simulink model "FMS22"  (R2018b)
settings: configuration reference "fms_config" (kept outside this file)
values from neighbouring files (symbols this model uses):
  FMS_EXPORT = Simulink.Parameter(FMS_EXPORT_VALUE)    [fms_model_init.m]
  FMS_PARAM = Simulink.Parameter(FMS_PARAM_VALUE)    [fms_model_init.m]
undefined symbols (not defined in the file or in its folder): actuator_cmd, ControlMode, ctrl_mode, DiscIntNeverNeededParam, mode, p_cmd, phi_cmd, psi_rate_cmd, q_cmd, r_cmd, reset, status, theta_cmd, throttle_cmd, u_cmd, v_cmd, VehicleMode, VehicleStatus, w_cmd
libraries: FMT_Model_Lib x18, simulink x16
(part 1 of 4)
settings Model: Creator=jiachi  LastModifiedBy=jiachi
settings ConfigSetRef: SourceLocation=Base Workspace

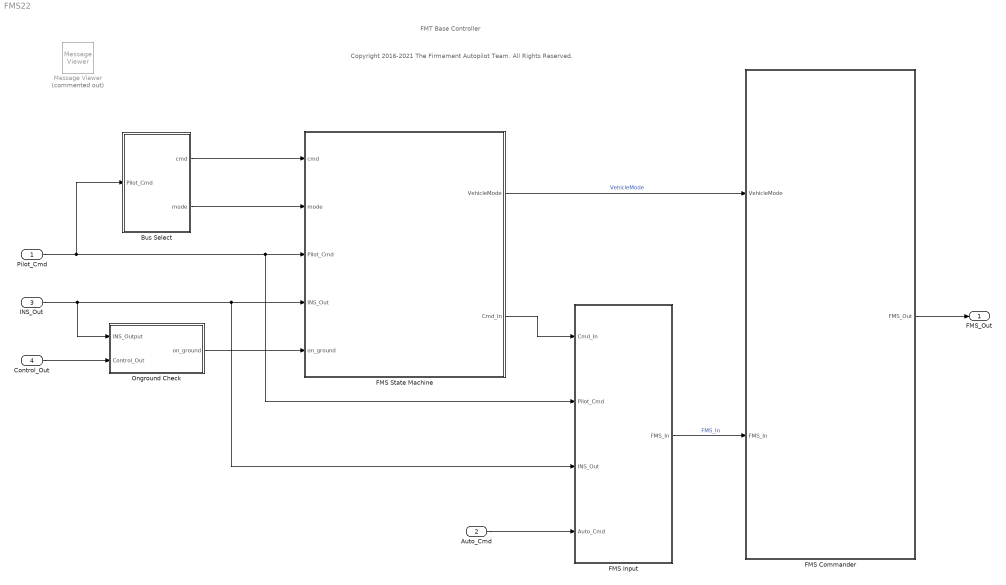
== system FMS22 ==
  note: FMT Base Controller
  note: Copyright 2016-2021 The Firmament Autopilot Team. All Rights Reserved.
  Pilot_Cmd : Inport  OutDataTypeStr=Bus: Pilot_Cmd_Bus
  Auto_Cmd : Inport  Port=2  OutDataTypeStr=Bus: Auto_Cmd_Bus
  INS_Out : Inport  Port=3  OutDataTypeStr=Bus: INS_Out_Bus
  Control_Out : Inport  Port=4  OutDataTypeStr=Bus: Control_Out_Bus
  Bus Select : Subsystem
  FMS Commander : Subsystem  TreatAsAtomicUnit=on
  FMS Input : Subsystem  TreatAsAtomicUnit=on
  FMS State Machine : Stateflow chart  TreatAsAtomicUnit=on
  Message Viewer : MessageViewer  Commented=on  SavedRootId=#
  Onground Check : Subsystem
  FMS_Out : Outport  OutDataTypeStr=Bus: FMS_Out_Bus
  wires:
  Pilot_Cmd/1 -> FMS State Machine/3(Pilot_Cmd), FMS Input/2(Pilot_Cmd), Bus Select/1(Pilot_Cmd)
  INS_Out/1 -> FMS Input/3(INS_Out), FMS State Machine/4(INS_Out), Onground Check/1(INS_Output)
  Control_Out/1 -> Onground Check/2(Control_Out)
  Onground Check/1(on_ground) -> FMS State Machine/5(on_ground)
  FMS State Machine/1(" VehicleMode") -> FMS Commander/1(VehicleMode)  "VehicleMode"
  FMS Input/1(FMS_In) -> FMS Commander/2(FMS_In)  "FMS_In"
  Auto_Cmd/1 -> FMS Input/4(Auto_Cmd)
  FMS Commander/1(FMS_Out) -> FMS_Out/1
  FMS State Machine/2(Cmd_In) -> FMS Input/1(Cmd_In)
  Bus Select/1(cmd) -> FMS State Machine/1(cmd)
  Bus Select/2(mode) -> FMS State Machine/2(mode)

== system FMS22/Bus Select ==
  Pilot_Cmd : Inport
  Bus Selector : BusSelector  OutputSignals=cmd_1,mode
  Data Type Conversion : DataTypeConversion  OutDataTypeStr=Enum: FMS_Cmd
  Data Type Conversion1 : DataTypeConversion  OutDataTypeStr=Enum: PilotMode
  cmd : Outport
  mode : Outport  Port=2
  wires:
  Data Type Conversion1/1 -> mode/1
  Pilot_Cmd/1 -> Bus Selector/1
  Bus Selector/1 -> Data Type Conversion/1  "<cmd_1>"
  Bus Selector/2 -> Data Type Conversion1/1  "<mode>"
  Data Type Conversion/1 -> cmd/1

== system FMS22/FMS Commander ==
  In Bus Element1 : Inport  PortName=VehicleMode
  In Bus Element2 : Inport  PortName=VehicleMode
  In Bus Element : Inport  Port=2  PortName=FMS_In
  Arm : Subsystem  TreatAsAtomicUnit=on
  Bus Assignment : BusAssignment  AssignedSignals=timestamp
  Disarm : Subsystem  TreatAsAtomicUnit=on
  Merge : Merge  Inputs=3
  Standby : Subsystem  TreatAsAtomicUnit=on
  Switch Case : SwitchCase  CaseConditions={[VehicleMode.Disarm,VehicleMode.None], VehicleMode.Standby}
  timestamp : Subsystem  mask{sample_time=FMS_EXPORT.period}
      mask prompts: sample_time "sample time (ms)"
  FMS_Out : Outport
  wires:
  Switch Case/1 -> Disarm/Action
  Merge/1 -> Bus Assignment/1
  Switch Case/2 -> Standby/Action
  Switch Case/3 -> Arm/Action
  Disarm/1(FMS_Out) -> Merge/1
  Standby/1(FMS_Out) -> Merge/2
  Arm/1(FMS_Out) -> Merge/3
  In Bus Element/1 -> Arm/2(FMS_In)
  In Bus Element1/1 -> Switch Case/1
  In Bus Element2/1 -> Arm/1(VehicleMode)
  timestamp/1(timestamp_ms) -> Bus Assignment/2
  Bus Assignment/1 -> FMS_Out/1

== system FMS22/FMS Input ==
  Cmd_In : Inport
  Pilot_Cmd : Inport  Port=2
  INS_Out : Inport  Port=3
  Auto_Cmd : Inport  Port=4
  Bus Creator : BusCreator  Inputs=4
  Signal Copy{,1..3} (4 alike) : SignalConversion  OverrideOpt=off
  FMS_In : Outport
  wires:
  Bus Creator/1 -> FMS_In/1
  Pilot_Cmd/1 -> Signal Copy2/1
  Auto_Cmd/1 -> Signal Copy/1
  INS_Out/1 -> Signal Copy1/1
  Signal Copy2/1 -> Bus Creator/1  "Pilot_Cmd"
  Signal Copy/1 -> Bus Creator/2  "Auto_Cmd"
  Signal Copy1/1 -> Bus Creator/3  "INS_Out"
  Cmd_In/1 -> Signal Copy3/1
  Signal Copy3/1 -> Bus Creator/4  "Cmd_In"

== system FMS22/Onground Check ==
  INS_Output : Inport
  Control_Out : Inport  Port=2
  Bus Selector1 : BusSelector  OutputSignals=actuator_cmd
  Bus Selector3 : BusSelector  OutputSignals=ax,ay,az
  Compare To Constant : simulink/Logic and Bit Operations/Compare To Constant  relop=<  const=1200  OutDataTypeStr=boolean
  Constant : Constant  Value=4  OutDataTypeStr=uint16
  Divide : Product  Inputs=*/
  First Order LPF : FMT_Model_Lib/Filter/First Order LPF  fc=1/(2*pi*0.5)
      settings: SourceProductName=FMT Toolbox
  First Order LPF2 : FMT_Model_Lib/Filter/First Order LPF  fc=1/(2*pi*0.1)
      settings: SourceProductName=FMT Toolbox
  Interval Test : simulink/Logic and Bit Operations/Interval Test  IntervalClosedRight=on  uplimit=[0.5, 0.5, -9.806+0.5]  IntervalClosedLeft=on  lowlimit=[-0.5, -0.5, -9.806-0.5]  OutDataTypeStr=boolean
  Logical Operator : Logic  Inputs=1  AllPortsSameDT=off  OutDataTypeStr=boolean
  Logical Operator1 : Logic  AllPortsSameDT=off  OutDataTypeStr=boolean
  Matrix Concatenate3 : Concatenate  NumInputs=3  ConcatenateDimension=2
  Selector : Selector  InputPortWidth=16  IndexOptions=Index vector (dialog)  Indices=[1:4]  OutputSizes=1
  Sum of Elements : Sum  Inputs=+
  on_ground : Outport
  wires:
  Bus Selector3/2 -> Matrix Concatenate3/2  "<ay>"
  Compare To Constant/1 -> Logical Operator1/2
  Bus Selector3/3 -> Matrix Concatenate3/3  "<az>"
  Bus Selector1/1 -> Selector/1  "<actuator_cmd>"
  Bus Selector3/1 -> Matrix Concatenate3/1  "<ax>"
  Selector/1 -> Sum of Elements/1
  INS_Output/1 -> Bus Selector3/1
  Control_Out/1 -> Bus Selector1/1
  Matrix Concatenate3/1 -> First Order LPF/1
  Interval Test/1 -> Logical Operator/1
  Sum of Elements/1 -> Divide/1
  Constant/1 -> Divide/2
  First Order LPF/1 -> Interval Test/1
  Divide/1 -> First Order LPF2/1
  First Order LPF2/1 -> Compare To Constant/1
  Logical Operator/1 -> Logical Operator1/1
  Logical Operator1/1 -> on_ground/1

== system FMS22/FMS Commander/Arm ==
  In Bus Element{2..5} (4 alike) : Inport  PortName=VehicleMode
  In Bus Element{,1,6..7} (4 alike) : Inport  Port=2  PortName=FMS_In
  Action Port : ActionPort  InitializeStates=reset  ActionType=default
  Assist : Subsystem  TreatAsAtomicUnit=on
  Auto : Subsystem  TreatAsAtomicUnit=on
  Manual : Subsystem  TreatAsAtomicUnit=on
  Merge : Merge  Inputs=4
  SubMode : Subsystem  TreatAsAtomicUnit=on
  Switch Case : SwitchCase  CaseConditions={[VehicleMode.Land,VehicleMode.Return,VehicleMode.Takeoff,VehicleMode.Hold], [VehicleMode.Offboard,VehicleMode.Mission],[VehicleMode.Acro,VehicleMode.Stabilize,VehicleMode.Altitude,VehicleMode.Position],VehicleMode.Manual}  ShowDefaultCase=off
  FMS_Out : Outport
  wires:
  Merge/1 -> FMS_Out/1
  Switch Case/1 -> SubMode/Action
  Switch Case/2 -> Auto/Action
  Switch Case/3 -> Assist/Action
  Switch Case/4 -> Manual/Action
  SubMode/1(FMS_Out) -> Merge/1
  Auto/1(FMS_Out) -> Merge/2
  Assist/1(FMS_Out) -> Merge/3
  Manual/1(FMS_Out) -> Merge/4
  In Bus Element/1 -> SubMode/2(FMS_In)
  In Bus Element1/1 -> Assist/2(FMS_In)
  In Bus Element2/1 -> Switch Case/1
  In Bus Element3/1 -> SubMode/1(VehicleMode)
  In Bus Element4/1 -> Assist/1(VehicleMode)
  In Bus Element5/1 -> Auto/1(VehicleMode)
  In Bus Element6/1 -> Auto/2(FMS_In)
  In Bus Element7/1 -> Manual/1(FMS_In)

== system FMS22/FMS Commander/Disarm ==
  Action Port : ActionPort  InitializeStates=reset  ActionType=case
  Bus Assignment : BusAssignment  AssignedSignals=reset,status,mode,actuator_cmd
  Constant : Constant  Value=0  OutDataTypeStr=Bus: FMS_Out_Bus
  Constant1 : Constant  Value=VehicleStatus.Disarm
  Constant2 : Constant  OutDataTypeStr=Inherit: Inherit via back propagation
  Constant3 : Constant  Value=[1000;1000;1000;1000]  VectorParams1D=off  OutDataTypeStr=Inherit: Inherit via back propagation
  Constant4 : Constant  Value=zeros(12,1)  OutDataTypeStr=Inherit: Inherit via back propagation
  Constant5 : Constant  Value=VehicleMode.Disarm
  Data Type Conversion : DataTypeConversion
  Data Type Conversion1 : DataTypeConversion
  Mux : Mux  Inputs=2
  FMS_Out : Outport
  wires:
  Mux/1 -> Bus Assignment/5
  Constant4/1 -> Mux/2
  Constant3/1 -> Mux/1
  Constant1/1 -> Data Type Conversion/1
  Constant2/1 -> Bus Assignment/2
  Bus Assignment/1 -> FMS_Out/1
  Constant/1 -> Bus Assignment/1
  Constant5/1 -> Data Type Conversion1/1
  Data Type Conversion/1 -> Bus Assignment/3
  Data Type Conversion1/1 -> Bus Assignment/4

== system FMS22/FMS Commander/Standby ==
  Action Port : ActionPort  InitializeStates=reset  ActionType=case
  Bus Assignment : BusAssignment  AssignedSignals=reset,status,mode,actuator_cmd
  Constant : Constant  Value=0  OutDataTypeStr=Bus: FMS_Out_Bus
  Constant1 : Constant  Value=VehicleStatus.Standby
  Constant2 : Constant  OutDataTypeStr=Inherit: Inherit via back propagation
  Constant3 : Constant  Value=[1150;1150;1150;1150]  VectorParams1D=off  OutDataTypeStr=Inherit: Inherit via back propagation
  Constant4 : Constant  Value=zeros(12,1)  OutDataTypeStr=Inherit: Inherit via back propagation
  Constant5 : Constant  Value=VehicleMode.Standby
  Data Type Conversion1 : DataTypeConversion
  Data Type Conversion2 : DataTypeConversion
  Mux : Mux  Inputs=2
  FMS_Out : Outport
  wires:
  Constant/1 -> Bus Assignment/1
  Bus Assignment/1 -> FMS_Out/1
  Constant2/1 -> Bus Assignment/2
  Constant1/1 -> Data Type Conversion2/1
  Constant3/1 -> Mux/1
  Constant4/1 -> Mux/2
  Constant5/1 -> Data Type Conversion1/1
  Data Type Conversion2/1 -> Bus Assignment/3
  Mux/1 -> Bus Assignment/5
  Data Type Conversion1/1 -> Bus Assignment/4

== system FMS22/FMS Commander/timestamp ==
  Constant : Constant  Value=sample_time
  Data Type Conversion : DataTypeConversion  OutDataTypeStr=uint32
  Discrete-Time Integrator : DiscreteIntegrator  IntegratorMethod=Accumulation: Forward Euler  SampleTime=-1  ICPrevOutput=DiscIntNeverNeededParam  ICPrevScaledInput=DiscIntNeverNeededParam
  timestamp_ms : Outport
  wires:
  Discrete-Time Integrator/1 -> Data Type Conversion/1
  Constant/1 -> Discrete-Time Integrator/1
  Data Type Conversion/1 -> timestamp_ms/1

== system FMS22/FMS Commander/Arm/Assist ==
  VehicleMode : Inport
  In Bus Element{1..4} (4 alike) : Inport  Port=2  PortName=FMS_In
  Action Port : ActionPort  InitializeStates=reset  ActionType=case
  Acro : Subsystem
      settings: UndoDeleteFcn=Stateflow.SLINSF.SimulinkMan.restorePreDeleteFcn  PreDeleteFcn=Stateflow.SLINSF.SimulinkMan.removePreDeleteFcn
  Altitude : Subsystem
      settings: UndoDeleteFcn=Stateflow.SLINSF.SimulinkMan.restorePreDeleteFcn  PreDeleteFcn=Stateflow.SLINSF.SimulinkMan.removePreDeleteFcn
  Merge : Merge  Inputs=4
  Position : Subsystem
      settings: UndoDeleteFcn=Stateflow.SLINSF.SimulinkMan.restorePreDeleteFcn  PreDeleteFcn=Stateflow.SLINSF.SimulinkMan.removePreDeleteFcn
  Stabilize : Subsystem
      settings: UndoDeleteFcn=Stateflow.SLINSF.SimulinkMan.restorePreDeleteFcn  PreDeleteFcn=Stateflow.SLINSF.SimulinkMan.removePreDeleteFcn
  Switch Case : SwitchCase  CaseConditions={VehicleMode.Acro,VehicleMode.Stabilize,VehicleMode.Altitude,VehicleMode.Position}  ShowDefaultCase=off
  FMS_Out : Outport
  wires:
  VehicleMode/1 -> Switch Case/1
  In Bus Element1/1 -> Position/1(FMS_In)
  Switch Case/4 -> Position/Action
  Switch Case/3 -> Altitude/Action
  In Bus Element2/1 -> Altitude/1(FMS_In)
  Switch Case/2 -> Stabilize/Action
  In Bus Element3/1 -> Stabilize/1(FMS_In)
  In Bus Element4/1 -> Acro/1(FMS_In)
  Switch Case/1 -> Acro/Action
  Acro/1(FMS_Out) -> Merge/1
  Stabilize/1(FMS_Out) -> Merge/2
  Altitude/1(FMS_Out) -> Merge/3
  Position/1(FMS_Out) -> Merge/4
  Merge/1 -> FMS_Out/1

== system FMS22/FMS Commander/Arm/Auto ==
  In Bus Element5 : Inport  PortName=VehicleMode
  In Bus Element6 : Inport  Port=2  PortName=FMS_In
  In Bus Element1 : Inport  Port=2  PortName=FMS_In
  Action Port : ActionPort  InitializeStates=reset  ActionType=case
  Merge : Merge
  Mission : Subsystem
      settings: UndoDeleteFcn=Stateflow.SLINSF.SimulinkMan.restorePreDeleteFcn  PreDeleteFcn=Stateflow.SLINSF.SimulinkMan.removePreDeleteFcn
  Offboard : Subsystem
      settings: UndoDeleteFcn=Stateflow.SLINSF.SimulinkMan.restorePreDeleteFcn  PreDeleteFcn=Stateflow.SLINSF.SimulinkMan.removePreDeleteFcn
  Switch Case : SwitchCase  CaseConditions={VehicleMode.Offboard,VehicleMode.Mission}  ShowDefaultCase=off
  FMS_Out : Outport
  wires:
  Merge/1 -> FMS_Out/1
  In Bus Element5/1 -> Switch Case/1
  In Bus Element6/1 -> Offboard/1(FMS_In)
  Switch Case/1 -> Offboard/Action
  In Bus Element1/1 -> Mission/1(FMS_In)
  Switch Case/2 -> Mission/Action
  Offboard/1(FMS_Out) -> Merge/1
  Mission/1(FMS_Out) -> Merge/2

== system FMS22/FMS Commander/Arm/Manual ==
  In Bus Element7 : Inport  PortName=FMS_In
  Action Port : ActionPort  InitializeStates=reset  ActionType=case
  Bus Assignment : BusAssignment  AssignedSignals=reset,status,mode
  Constant : Constant  Value=0  OutDataTypeStr=Bus: FMS_Out_Bus
  Constant1 : Constant  Value=VehicleStatus.Disarm
  Constant2 : Constant  OutDataTypeStr=Inherit: Inherit via back propagation
  Constant5 : Constant  Value=VehicleMode.Manual
  Data Type Conversion : DataTypeConversion
  Data Type Conversion1 : DataTypeConversion
  Terminator : Terminator
  FMS_Out : Outport
  wires:
  Data Type Conversion1/1 -> Bus Assignment/4
  Data Type Conversion/1 -> Bus Assignment/3
  Constant5/1 -> Data Type Conversion1/1
  Constant/1 -> Bus Assignment/1
  Bus Assignment/1 -> FMS_Out/1
  Constant2/1 -> Bus Assignment/2
  Constant1/1 -> Data Type Conversion/1
  In Bus Element7/1 -> Terminator/1

== system FMS22/FMS Commander/Arm/SubMode ==
  In Bus Element : Inport  PortName=VehicleMode
  In Bus Element{1..4} (4 alike) : Inport  Port=2  PortName=FMS_In
  Action Port : ActionPort  InitializeStates=reset  ActionType=case
  Hold : Subsystem
      settings: UndoDeleteFcn=Stateflow.SLINSF.SimulinkMan.restorePreDeleteFcn  PreDeleteFcn=Stateflow.SLINSF.SimulinkMan.removePreDeleteFcn
  Land : Subsystem
      settings: UndoDeleteFcn=Stateflow.SLINSF.SimulinkMan.restorePreDeleteFcn  PreDeleteFcn=Stateflow.SLINSF.SimulinkMan.removePreDeleteFcn
  Merge : Merge  Inputs=4
  Return : Subsystem
      settings: UndoDeleteFcn=Stateflow.SLINSF.SimulinkMan.restorePreDeleteFcn  PreDeleteFcn=Stateflow.SLINSF.SimulinkMan.removePreDeleteFcn
  Switch Case : SwitchCase  CaseConditions={VehicleMode.Takeoff, VehicleMode.Land, VehicleMode.Return,VehicleMode.Hold}  ShowDefaultCase=off
  Takeoff : Subsystem
      settings: UndoDeleteFcn=Stateflow.SLINSF.SimulinkMan.restorePreDeleteFcn  PreDeleteFcn=Stateflow.SLINSF.SimulinkMan.removePreDeleteFcn
  FMS_Out : Outport
  wires:
  Merge/1 -> FMS_Out/1
  In Bus Element/1 -> Switch Case/1
  In Bus Element1/1 -> Land/1(FMS_In)
  Land/1(FMS_Out) -> Merge/2
  Switch Case/2 -> Land/Action
  Switch Case/1 -> Takeoff/Action
  In Bus Element2/1 -> Takeoff/1(FMS_In)
  Takeoff/1(FMS_Out) -> Merge/1
  Switch Case/3 -> Return/Action
  In Bus Element3/1 -> Return/1(FMS_In)
  Return/1(FMS_Out) -> Merge/3
  Hold/1(FMS_Out) -> Merge/4
  In Bus Element4/1 -> Hold/1(FMS_In)
  Switch Case/4 -> Hold/Action

== system FMS22/FMS Commander/Arm/Assist/Acro ==
  FMS_In : Inport
  Action Port : ActionPort  InitializeStates=reset  ActionType=case
      settings: CopyFcn=Stateflow.SLINSF.SimulinkMan.removeBlockPreDeleteFcn
  Angular Rate Command : Subsystem
  Bus Assignment : BusAssignment  AssignedSignals=status,mode,ctrl_mode,p_cmd,q_cmd,r_cmd,throttle_cmd
  Constant : Constant  Value=0  OutDataTypeStr=Bus: FMS_Out_Bus
  Constant1 : Constant  Value=VehicleMode.Acro
  Constant2 : Constant  Value=ControlMode.Acro
  Constant5 : Constant  Value=VehicleStatus.Arm
  Data Type Conversion : DataTypeConversion
  Data Type Conversion1 : DataTypeConversion
  Data Type Conversion2 : DataTypeConversion
  Throttle Command : Subsystem
  FMS_Out : Outport
  wires:
  Data Type Conversion2/1 -> Bus Assignment/4
  Constant2/1 -> Data Type Conversion2/1
  Data Type Conversion1/1 -> Bus Assignment/3
  Constant1/1 -> Data Type Conversion1/1
  Data Type Conversion/1 -> Bus Assignment/2
  Bus Assignment/1 -> FMS_Out/1
  Throttle Command/1(throttle_cmd) -> Bus Assignment/8
  Constant/1 -> Bus Assignment/1
  Constant5/1 -> Data Type Conversion/1
  Angular Rate Command/1(p_cmd_radPs) -> Bus Assignment/5
  Angular Rate Command/2(q_cmd_radPs) -> Bus Assignment/6
  Angular Rate Command/3(r_cmd_radPs) -> Bus Assignment/7
  FMS_In/1 -> Throttle Command/1(FMS_In), Angular Rate Command/1(FMS_In)

== system FMS22/FMS Commander/Arm/Assist/Altitude ==
  In Bus Element1 : Inport  PortName=FMS_In
  Action Port : ActionPort  InitializeStates=reset  ActionType=case
      settings: CopyFcn=Stateflow.SLINSF.SimulinkMan.removeBlockPreDeleteFcn
  Altitude Command : Subsystem
  Attitude Command : Subsystem
  Bus Assignment : BusAssignment  AssignedSignals=status,mode,ctrl_mode,phi_cmd,theta_cmd,psi_rate_cmd,w_cmd
  Constant : Constant  Value=0  OutDataTypeStr=Bus: FMS_Out_Bus
  Constant1 : Constant  Value=VehicleMode.Altitude
  Constant2 : Constant  Value=ControlMode.ALTCTL
  Constant5 : Constant  Value=VehicleStatus.Arm
  Data Type Conversion1 : DataTypeConversion
  Data Type Conversion2 : DataTypeConversion
  Data Type Conversion3 : DataTypeConversion
  Heading Command : Subsystem
  FMS_Out : Outport
  wires:
  Constant5/1 -> Data Type Conversion1/1
  Constant/1 -> Bus Assignment/1
  Heading Command/1(psi_rate_cmd_radPs) -> Bus Assignment/7
  Altitude Command/1(w_cmd_mPs) -> Bus Assignment/8
  Attitude Command/1(phi_cmd_radPs) -> Bus Assignment/5
  Attitude Command/2(theta_cmd_radPs) -> Bus Assignment/6
  Bus Assignment/1 -> FMS_Out/1
  Data Type Conversion1/1 -> Bus Assignment/2
  Constant1/1 -> Data Type Conversion2/1
  Data Type Conversion2/1 -> Bus Assignment/3
  Data Type Conversion3/1 -> Bus Assignment/4
  Constant2/1 -> Data Type Conversion3/1
  In Bus Element1/1 -> Heading Command/1(FMS_In), Altitude Command/1(FMS_In), Attitude Command/1(FMS_In)

== system FMS22/FMS Commander/Arm/Assist/Position ==
  FMS_In : Inport
  Action Port : ActionPort  InitializeStates=reset  ActionType=case
      settings: CopyFcn=Stateflow.SLINSF.SimulinkMan.removeBlockPreDeleteFcn
  Altitude Command : Subsystem
  Bus Assignment : BusAssignment  AssignedSignals=status,mode,ctrl_mode,psi_rate_cmd,u_cmd,v_cmd,w_cmd
  Constant : Constant  Value=0  OutDataTypeStr=Bus: FMS_Out_Bus
  Constant1 : Constant  Value=VehicleMode.Position
  Constant2 : Constant  Value=ControlMode.POSCTL
  Constant5 : Constant  Value=VehicleStatus.Arm
  Data Type Conversion : DataTypeConversion
  Data Type Conversion1 : DataTypeConversion
  Data Type Conversion2 : DataTypeConversion
  Heading Command : Subsystem
  Position Command : Subsystem
  FMS_Out : Outport
  wires:
  Bus Assignment/1 -> FMS_Out/1
  Altitude Command/1(w_cmd_mPs) -> Bus Assignment/8
  Constant/1 -> Bus Assignment/1
  Position Command/1(u_cmd_mPs) -> Bus Assignment/6
  Constant5/1 -> Data Type Conversion/1
  Position Command/2(v_cmd_mPs) -> Bus Assignment/7
  Heading Command/1(psi_rate_cmd_radPs) -> Bus Assignment/5
  Data Type Conversion/1 -> Bus Assignment/2
  Constant1/1 -> Data Type Conversion1/1
  Data Type Conversion1/1 -> Bus Assignment/3
  Constant2/1 -> Data Type Conversion2/1
  Data Type Conversion2/1 -> Bus Assignment/4
  FMS_In/1 -> Heading Command/1(FMS_In), Altitude Command/1(FMS_In), Position Command/1(FMS_In)

== system FMS22/FMS Commander/Arm/Assist/Stabilize ==
  FMS_In : Inport
  Action Port : ActionPort  InitializeStates=reset  ActionType=case
      settings: CopyFcn=Stateflow.SLINSF.SimulinkMan.removeBlockPreDeleteFcn
  Attitude Command : Subsystem
  Bus Assignment : BusAssignment  AssignedSignals=status,mode,ctrl_mode,phi_cmd,theta_cmd,psi_rate_cmd,throttle_cmd
  Constant : Constant  Value=0  OutDataTypeStr=Bus: FMS_Out_Bus
  Constant1 : Constant  Value=VehicleMode.Stabilize
  Constant2 : Constant  Value=ControlMode.Stabilize
  Constant5 : Constant  Value=VehicleStatus.Arm
  Data Type Conversion : DataTypeConversion
  Data Type Conversion1 : DataTypeConversion
  Data Type Conversion2 : DataTypeConversion
  Heading Command : Subsystem
  Throttle Command : Subsystem
  FMS_Out : Outport
  wires:
  Constant5/1 -> Data Type Conversion/1
  Heading Command/1(psi_rate_cmd_radPs) -> Bus Assignment/7
  Constant/1 -> Bus Assignment/1
  Attitude Command/1(phi_cmd_radPs) -> Bus Assignment/5
  Throttle Command/1(throttle_cmd) -> Bus Assignment/8
  Attitude Command/2(theta_cmd_radPs) -> Bus Assignment/6
  FMS_In/1 -> Throttle Command/1(FMS_In), Heading Command/1(FMS_In), Attitude Command/1(FMS_In)
  Bus Assignment/1 -> FMS_Out/1
  Data Type Conversion/1 -> Bus Assignment/2
  Constant1/1 -> Data Type Conversion1/1
  Data Type Conversion1/1 -> Bus Assignment/3
  Constant2/1 -> Data Type Conversion2/1
  Data Type Conversion2/1 -> Bus Assignment/4

== system FMS22/FMS Commander/Arm/Auto/Mission ==
  FMS_In : Inport
  Action Port : ActionPort  InitializeStates=reset  ActionType=case
      settings: CopyFcn=Stateflow.SLINSF.SimulinkMan.removeBlockPreDeleteFcn
  Bus Assignment : BusAssignment  AssignedSignals=status,mode
  Constant : Constant  Value=0  OutDataTypeStr=Bus: FMS_Out_Bus
  Constant1 : Constant  Value=VehicleStatus.Disarm
  Constant2 : Constant  Value=VehicleMode.Mission
  Data Type Conversion : DataTypeConversion
  Data Type Conversion1 : DataTypeConversion
  Terminator : Terminator
  FMS_Out : Outport
  wires:
  Bus Assignment/1 -> FMS_Out/1
  Constant/1 -> Bus Assignment/1
  FMS_In/1 -> Terminator/1
  Constant1/1 -> Data Type Conversion/1
  Data Type Conversion/1 -> Bus Assignment/2
  Constant2/1 -> Data Type Conversion1/1
  Data Type Conversion1/1 -> Bus Assignment/3

== system FMS22/FMS Commander/Arm/Auto/Offboard ==
  FMS_In : Inport
  Action Port : ActionPort  InitializeStates=reset  ActionType=case
      settings: CopyFcn=Stateflow.SLINSF.SimulinkMan.removeBlockPreDeleteFcn
  Bus Assignment : BusAssignment  AssignedSignals=status,mode
  Constant : Constant  Value=0  OutDataTypeStr=Bus: FMS_Out_Bus
  Constant1 : Constant  Value=VehicleStatus.Disarm
  Constant2 : Constant  Value=VehicleMode.Offboard
  Data Type Conversion : DataTypeConversion
  Data Type Conversion1 : DataTypeConversion
  Terminator : Terminator
  FMS_Out : Outport
  wires:
  Bus Assignment/1 -> FMS_Out/1
  Constant/1 -> Bus Assignment/1
  FMS_In/1 -> Terminator/1
  Constant1/1 -> Data Type Conversion/1
  Data Type Conversion/1 -> Bus Assignment/2
  Constant2/1 -> Data Type Conversion1/1
  Data Type Conversion1/1 -> Bus Assignment/3

== system FMS22/FMS Commander/Arm/SubMode/Hold ==
  FMS_In : Inport
  Action Port : ActionPort  InitializeStates=reset  ActionType=case
      settings: CopyFcn=Stateflow.SLINSF.SimulinkMan.removeBlockPreDeleteFcn
  Altitude Command : Subsystem
  Bus Assignment : BusAssignment  AssignedSignals=status,mode,ctrl_mode,psi_rate_cmd,u_cmd,v_cmd,w_cmd
  Constant : Constant  Value=0  OutDataTypeStr=Bus: FMS_Out_Bus
  Constant1 : Constant  Value=VehicleMode.Hold
  Constant2 : Constant  Value=ControlMode.POSCTL
  Constant5 : Constant  Value=VehicleStatus.Arm
  Data Type Conversion : DataTypeConversion
  Data Type Conversion1 : DataTypeConversion
  Data Type Conversion2 : DataTypeConversion
  Heading Command : Subsystem
  Position Command : Subsystem
  FMS_Out : Outport
  wires:
  Bus Assignment/1 -> FMS_Out/1
  Altitude Command/1(w_cmd_mPs) -> Bus Assignment/8
  Constant/1 -> Bus Assignment/1
  Position Command/1(u_cmd_mPs) -> Bus Assignment/6
  Constant5/1 -> Data Type Conversion/1
  Position Command/2(v_cmd_mPs) -> Bus Assignment/7
  Heading Command/1(psi_rate_cmd_radPs) -> Bus Assignment/5
  Data Type Conversion/1 -> Bus Assignment/2
  Constant1/1 -> Data Type Conversion1/1
  Data Type Conversion1/1 -> Bus Assignment/3
  Constant2/1 -> Data Type Conversion2/1
  Data Type Conversion2/1 -> Bus Assignment/4
  FMS_In/1 -> Heading Command/1(FMS_In), Altitude Command/1(FMS_In), Position Command/1(FMS_In)

== system FMS22/FMS Commander/Arm/SubMode/Land ==
  FMS_In : Inport
  Action Port : ActionPort  InitializeStates=reset  ActionType=case
      settings: CopyFcn=Stateflow.SLINSF.SimulinkMan.removeBlockPreDeleteFcn
  Bus Assignment1 : BusAssignment  AssignedSignals=status,mode,ctrl_mode,psi_rate_cmd,u_cmd,v_cmd,w_cmd
  Bus Selector : BusSelector  OutputSignals=Cmd_In.p_land
  Constant : Constant  Value=0  OutDataTypeStr=Inherit: Inherit via back propagation
  Constant1 : Constant  Value=0  OutDataTypeStr=Bus: FMS_Out_Bus
  Constant2 : Constant  Value=ControlMode.POSCTL
  Constant3 : Constant  Value=VehicleMode.Land
  Constant4 : Constant  Value=0.5  OutDataTypeStr=Inherit: Inherit via back propagation
  Constant6 : Constant  Value=VehicleStatus.Arm
  Data Type Conversion : DataTypeConversion
  Data Type Conversion1 : DataTypeConversion
  Data Type Conversion2 : DataTypeConversion
  Position Command : Subsystem
  Reshape : Reshape  OutputDimensionality=Customize  OutputDimensions=[2,1]
  FMS_Out : Outport
  wires:
  Reshape/1 -> Position Command/2(land_xy_R)
  Bus Assignment1/1 -> FMS_Out/1
  Constant1/1 -> Bus Assignment1/1
  FMS_In/1 -> Position Command/1(FMS_In), Bus Selector/1
  Constant4/1 -> Bus Assignment1/8
  Position Command/1(u_cmd_mPs) -> Bus Assignment1/6
  Position Command/2(v_cmd_mPs) -> Bus Assignment1/7
  Constant/1 -> Bus Assignment1/5
  Constant2/1 -> Data Type Conversion2/1
  Constant6/1 -> Data Type Conversion/1
  Data Type Conversion/1 -> Bus Assignment1/2
  Constant3/1 -> Data Type Conversion1/1
  Data Type Conversion1/1 -> Bus Assignment1/3
  Data Type Conversion2/1 -> Bus Assignment1/4
  Bus Selector/1 -> Reshape/1  "<p_land>"

== system FMS22/FMS Commander/Arm/SubMode/Return ==
  FMS_In : Inport
  Action Port : ActionPort  InitializeStates=reset  ActionType=case
      settings: CopyFcn=Stateflow.SLINSF.SimulinkMan.removeBlockPreDeleteFcn
  Bus Assignment1 : BusAssignment  AssignedSignals=status,mode,ctrl_mode,u_cmd,v_cmd,w_cmd,psi_rate_cmd
  Bus Selector : BusSelector  OutputSignals=INS_Out
  Constant1 : Constant  Value=VehicleMode.Return
  Constant2 : Constant  Value=0  OutDataTypeStr=Bus: FMS_Out_Bus
  Constant3 : Constant  Value=ControlMode.POSCTL
  Constant6 : Constant  Value=VehicleStatus.Arm
  Coordinate Points : Subsystem
  Data Type Conversion : DataTypeConversion
  Data Type Conversion1 : DataTypeConversion
  Data Type Conversion2 : DataTypeConversion
  Heading Commander : Subsystem
  L1 : Constant  Value=10  OutDataTypeStr=single
  Sum : Sum  Inputs=+-|
  Velocity Commander : Subsystem
  FMS_Out : Outport
  wires:
  Sum/1 -> Heading Commander/2(p1p2)
  Velocity Commander/1(u_cmd) -> Bus Assignment1/5
  Coordinate Points/2(p2) -> Sum/1, Velocity Commander/2(p2)
  Coordinate Points/3(p3) -> Velocity Commander/3(p3)
  Velocity Commander/3(w_cmd) -> Bus Assignment1/7
  L1/1 -> Velocity Commander/4(L1)
  Velocity Commander/2(v_cmd) -> Bus Assignment1/6
  Constant3/1 -> Data Type Conversion2/1
  Coordinate Points/1(p1) -> Velocity Commander/1(p1), Sum/2
  Constant2/1 -> Bus Assignment1/1
  Heading Commander/1(psi_rad_cmd) -> Bus Assignment1/8
  Bus Assignment1/1 -> FMS_Out/1
  FMS_In/1 -> Bus Selector/1, Heading Commander/1(FMS_In), Coordinate Points/1(FMS_In)
  Data Type Conversion/1 -> Bus Assignment1/2
  Constant6/1 -> Data Type Conversion/1
  Data Type Conversion1/1 -> Bus Assignment1/3
  Data Type Conversion2/1 -> Bus Assignment1/4
  Constant1/1 -> Data Type Conversion1/1
  Bus Selector/1 -> Velocity Commander/5(INS_Out)  "<INS_Out>"

== system FMS22/FMS Commander/Arm/SubMode/Takeoff ==
  FMS_In : Inport
  Action Port : ActionPort  InitializeStates=reset  ActionType=case
      settings: CopyFcn=Stateflow.SLINSF.SimulinkMan.removeBlockPreDeleteFcn
  Bus Assignment1 : BusAssignment  AssignedSignals=status,mode,ctrl_mode,psi_rate_cmd,u_cmd,v_cmd,w_cmd
  Constant : Constant  Value=0  OutDataTypeStr=Inherit: Inherit via back propagation
  Constant1 : Constant  Value=0  OutDataTypeStr=Bus: FMS_Out_Bus
  Constant2 : Constant  Value=ControlMode.POSCTL
  Constant3 : Constant  Value=VehicleMode.Takeoff
  Constant4 : Constant  Value=-0.5  OutDataTypeStr=Inherit: Inherit via back propagation
  Constant5 : Constant  Value=VehicleStatus.Arm
  Data Type Conversion : DataTypeConversion
  Data Type Conversion1 : DataTypeConversion
  Data Type Conversion2 : DataTypeConversion
  Demux : Demux  Outputs=2
  Hold Position : Subsystem
  FMS_Out : Outport
  wires:
  Constant5/1 -> Data Type Conversion/1
  Constant4/1 -> Bus Assignment1/8
  Demux/2 -> Bus Assignment1/7
  Demux/1 -> Bus Assignment1/6
  Constant/1 -> Bus Assignment1/5
  Constant2/1 -> Data Type Conversion2/1
  Hold Position/1(uv_cmd_mPs) -> Demux/1
  Constant1/1 -> Bus Assignment1/1
  FMS_In/1 -> Hold Position/1(FMS_In)
  Bus Assignment1/1 -> FMS_Out/1
  Data Type Conversion/1 -> Bus Assignment1/2
  Data Type Conversion1/1 -> Bus Assignment1/3
  Constant3/1 -> Data Type Conversion1/1
  Data Type Conversion2/1 -> Bus Assignment1/4

== system FMS22/FMS Commander/Arm/Assist/Acro/Angular Rate Command ==
  FMS_In : Inport
  Bus Selector : BusSelector  OutputSignals=Pilot_Cmd.stick_roll,Pilot_Cmd.stick_pitch,Pilot_Cmd.stick_yaw
  Gain : Gain  Gain=pi
  Gain1 : Gain  Gain=-pi
  Gain2 : Gain  Gain=pi/2
  p_cmd_radPs : Outport
  q_cmd_radPs : Outport  Port=2
  r_cmd_radPs : Outport  Port=3
  wires:
  FMS_In/1 -> Bus Selector/1
  Gain2/1 -> r_cmd_radPs/1
  Gain1/1 -> q_cmd_radPs/1
  Bus Selector/3 -> Gain2/1  "<stick_yaw>"
  Bus Selector/2 -> Gain1/1  "<stick_pitch>"
  Gain/1 -> p_cmd_radPs/1
  Bus Selector/1 -> Gain/1  "<stick_roll>"

== system FMS22/FMS Commander/Arm/Assist/Acro/Throttle Command ==
  FMS_In : Inport
  Add : Sum
  Bus Selector : BusSelector  OutputSignals=Pilot_Cmd.stick_throttle
  Constant4 : Constant  OutDataTypeStr=single
  Constant5 : Constant  Value=1000  OutDataTypeStr=uint32
  Gain2 : Gain  Gain=500  OutDataTypeStr=uint32
  Saturation : Saturate  UpperLimit=2  LowerLimit=0
  Sum : Sum  Inputs=|++
  throttle_cmd : Outport
  wires:
  Constant4/1 -> Sum/2
  Add/1 -> throttle_cmd/1
  Constant5/1 -> Add/2
  Bus Selector/1 -> Sum/1  "<stick_throttle>"
  Saturation/1 -> Gain2/1
  Sum/1 -> Saturation/1
  Gain2/1 -> Add/1
  FMS_In/1 -> Bus Selector/1

== system FMS22/FMS Commander/Arm/Assist/Altitude/Altitude Command ==
  FMS_In : Inport
  Controller : Subsystem
  Detect Movement : Subsystem
  w_cmd_mPs : Outport
  wires:
  Controller/1(w_cmd_mPs) -> w_cmd_mPs/1
  Detect Movement/1(motion_state) -> Controller/1(motion_state)
  FMS_In/1 -> Controller/2(FMS_In), Detect Movement/1(FMS_In)

== system FMS22/FMS Commander/Arm/Assist/Altitude/Attitude Command ==
  FMS_In : Inport
  Bus Selector : BusSelector  OutputSignals=Pilot_Cmd.stick_roll,Pilot_Cmd.stick_pitch
  DeadZone : Subsystem  mask{th=FMS_PARAM.ROLL_DZ}
      mask prompts: th "Threshold"
      mask Display: disp('Dead Zone')
  DeadZone2 : Subsystem  mask{th=FMS_PARAM.PITCH_DZ}
      mask prompts: th "Threshold"
      mask Display: disp('Dead Zone')
  Gain : Gain  Gain=FMS_PARAM.ROLL_PITCH_LIM
  Gain1 : Gain  Gain=-FMS_PARAM.ROLL_PITCH_LIM
  Phi_CMD_TD : Subsystem
  Theta_CMD_TD : Subsystem
  phi_cmd_radPs : Outport
  theta_cmd_radPs : Outport  Port=2
  wires:
  Bus Selector/2 -> DeadZone2/1(u)  "<stick_pitch>"
  Bus Selector/1 -> DeadZone/1(u)  "<stick_roll>"
  FMS_In/1 -> Bus Selector/1
  Theta_CMD_TD/1(v1) -> theta_cmd_radPs/1
  Phi_CMD_TD/1(v1) -> phi_cmd_radPs/1
  Gain1/1 -> Theta_CMD_TD/1(v)
  Gain/1 -> Phi_CMD_TD/1(v)
  DeadZone2/1(y) -> Gain1/1
  DeadZone/1(y) -> Gain/1

== system FMS22/FMS Commander/Arm/Assist/Altitude/Heading Command ==
  FMS_In : Inport
  Controller : Subsystem
  Detect Movement : Subsystem
  psi_rate_cmd_radPs : Outport
  wires:
  Controller/1(psi_rate_cmd_radPs) -> psi_rate_cmd_radPs/1
  Detect Movement/1(motion_state) -> Controller/1(motion_state)
  FMS_In/1 -> Controller/2(FMS_In), Detect Movement/1(FMS_In)

== system FMS22/FMS Commander/Arm/Assist/Position/Altitude Command ==
  FMS_In : Inport
  Controller : Subsystem
  Detect Movement : Subsystem
  w_cmd_mPs : Outport
  wires:
  Controller/1(w_cmd_mPs) -> w_cmd_mPs/1
  Detect Movement/1(motion_state) -> Controller/1(motion_state)
  FMS_In/1 -> Controller/2(FMS_In), Detect Movement/1(FMS_In)

== system FMS22/FMS Commander/Arm/Assist/Position/Heading Command ==
  FMS_In : Inport
  Controller : Subsystem
  Detect Movement : Subsystem
  psi_rate_cmd_radPs : Outport
  wires:
  Controller/1(psi_rate_cmd_radPs) -> psi_rate_cmd_radPs/1
  Detect Movement/1(motion_state) -> Controller/1(motion_state)
  FMS_In/1 -> Controller/2(FMS_In), Detect Movement/1(FMS_In)

== system FMS22/FMS Commander/Arm/Assist/Position/Position Command ==
  FMS_In : Inport
  Controller : Subsystem
  Demux : Demux  Outputs=2
  Detect Movement : Subsystem
  u_cmd_mPs : Outport
  v_cmd_mPs : Outport  Port=2
  wires:
  FMS_In/1 -> Controller/2(FMS_In), Detect Movement/1(FMS_In)
  Demux/2 -> v_cmd_mPs/1
  Demux/1 -> u_cmd_mPs/1
  Controller/1(uv_cmd_mPs) -> Demux/1
  Detect Movement/1(motion_state) -> Controller/1(motion_state)

== system FMS22/FMS Commander/Arm/Assist/Stabilize/Attitude Command ==
  FMS_In : Inport
  Bus Selector : BusSelector  OutputSignals=Pilot_Cmd.stick_roll,Pilot_Cmd.stick_pitch
  DeadZone : Subsystem  mask{th=FMS_PARAM.ROLL_DZ}
      mask prompts: th "Threshold"
      mask Display: disp('Dead Zone')
  DeadZone2 : Subsystem  mask{th=FMS_PARAM.PITCH_DZ}
      mask prompts: th "Threshold"
      mask Display: disp('Dead Zone')
  Gain : Gain  Gain=FMS_PARAM.ROLL_PITCH_LIM
  Gain1 : Gain  Gain=-FMS_PARAM.ROLL_PITCH_LIM
  Phi_CMD_TD : Subsystem
  Theta_CMD_TD : Subsystem
  phi_cmd_radPs : Outport
  theta_cmd_radPs : Outport  Port=2
  wires:
  Bus Selector/2 -> DeadZone2/1(u)  "<stick_pitch>"
  Bus Selector/1 -> DeadZone/1(u)  "<stick_roll>"
  FMS_In/1 -> Bus Selector/1
  Theta_CMD_TD/1(v1) -> theta_cmd_radPs/1
  Phi_CMD_TD/1(v1) -> phi_cmd_radPs/1
  Gain1/1 -> Theta_CMD_TD/1(v)
  Gain/1 -> Phi_CMD_TD/1(v)
  DeadZone2/1(y) -> Gain1/1
  DeadZone/1(y) -> Gain/1

== system FMS22/FMS Commander/Arm/Assist/Stabilize/Heading Command ==
  FMS_In : Inport
  Controller : Subsystem
  Detect Movement : Subsystem
  psi_rate_cmd_radPs : Outport
  wires:
  FMS_In/1 -> Detect Movement/1(FMS_In), Controller/2(FMS_In)
  Controller/1(psi_rate_cmd_radPs) -> psi_rate_cmd_radPs/1
  Detect Movement/1(motion_state) -> Controller/1(motion_state)

== system FMS22/FMS Commander/Arm/Assist/Stabilize/Throttle Command ==
  FMS_In : Inport
  Add : Sum
  Bus Selector : BusSelector  OutputSignals=Pilot_Cmd.stick_throttle
  Constant4 : Constant  OutDataTypeStr=single
  Constant5 : Constant  Value=1000  OutDataTypeStr=uint32
  Gain2 : Gain  Gain=500  OutDataTypeStr=uint32
  Saturation : Saturate  UpperLimit=2  LowerLimit=0
  Sum : Sum  Inputs=|++
  throttle_cmd : Outport
  wires:
  FMS_In/1 -> Bus Selector/1
  Gain2/1 -> Add/1
  Sum/1 -> Saturation/1
  Saturation/1 -> Gain2/1
  Bus Selector/1 -> Sum/1  "<stick_throttle>"
  Constant5/1 -> Add/2
  Add/1 -> throttle_cmd/1
  Constant4/1 -> Sum/2

== system FMS22/FMS Commander/Arm/SubMode/Hold/Altitude Command ==
  FMS_In : Inport
  Controller : Subsystem
  Detect Movement : Subsystem
  w_cmd_mPs : Outport
  wires:
  Controller/1(w_cmd_mPs) -> w_cmd_mPs/1
  Detect Movement/1(motion_state) -> Controller/1(motion_state)
  FMS_In/1 -> Controller/2(FMS_In), Detect Movement/1(FMS_In)

== system FMS22/FMS Commander/Arm/SubMode/Hold/Heading Command ==
  FMS_In : Inport
  Controller : Subsystem
  Detect Movement : Subsystem
  psi_rate_cmd_radPs : Outport
  wires:
  Controller/1(psi_rate_cmd_radPs) -> psi_rate_cmd_radPs/1
  Detect Movement/1(motion_state) -> Controller/1(motion_state)
  FMS_In/1 -> Controller/2(FMS_In), Detect Movement/1(FMS_In)

== system FMS22/FMS Commander/Arm/SubMode/Hold/Position Command ==
  FMS_In : Inport
  Controller : Subsystem
  Demux : Demux  Outputs=2
  Detect Movement : Subsystem
  u_cmd_mPs : Outport
  v_cmd_mPs : Outport  Port=2
  wires:
  FMS_In/1 -> Controller/2(FMS_In), Detect Movement/1(FMS_In)
  Demux/2 -> v_cmd_mPs/1
  Demux/1 -> u_cmd_mPs/1
  Controller/1(uv_cmd_mPs) -> Demux/1
  Detect Movement/1(motion_state) -> Controller/1(motion_state)

== system FMS22/FMS Commander/Arm/SubMode/Land/Position Command ==
  FMS_In : Inport
  land_xy_R : Inport  Port=2
  Demux : Demux  Outputs=2
  Position Control : Subsystem
  Saturation1 : Saturate  UpperLimit=FMS_PARAM.VEL_XY_LIM/5  LowerLimit=-FMS_PARAM.VEL_XY_LIM/5
  u_cmd_mPs : Outport
  v_cmd_mPs : Outport  Port=2
  wires:
  land_xy_R/1 -> Position Control/2(land_xy_R)
  Position Control/1(uv_cmd_mPs) -> Saturation1/1
  Demux/2 -> v_cmd_mPs/1
  Demux/1 -> u_cmd_mPs/1
  Saturation1/1 -> Demux/1
  FMS_In/1 -> Position Control/1(FMS_In)

== system FMS22/FMS Commander/Arm/SubMode/Return/Coordinate Points ==
  note: P1: path start point
      | P2: path end point
      | P3: vehicle point
  FMS_In : Inport
  Bus Selector : BusSelector  OutputSignals=INS_Out.x_R,INS_Out.y_R
  Bus Selector1 : BusSelector  OutputSignals=Cmd_In.p_return
  Delay : Delay  DelayLength=1  InitialConditionSource=Input port  InitialCondition=single([0 0])
      settings: InputPortMap=u0,p4
  Mux : Mux  Inputs=2
  Reshape : Reshape  OutputDimensionality=Customize  OutputDimensions=[2,1]
  Reshape1 : Reshape  OutputDimensionality=Customize  OutputDimensions=[2,1]
  Reshape2 : Reshape  OutputDimensionality=Customize  OutputDimensions=[2,1]
  p1 : Outport
  p2 : Outport  Port=2
  p3 : Outport  Port=3
  wires:
  Reshape2/1 -> p3/1
  Reshape1/1 -> p1/1
  Reshape/1 -> p2/1
  Bus Selector/2 -> Mux/2  "<y_R>"
  Bus Selector/1 -> Mux/1  "<x_R>"
  Mux/1 -> Reshape2/1, Delay/2
  Delay/1 -> Delay/1, Reshape1/1
  FMS_In/1 -> Bus Selector1/1, Bus Selector/1
  Bus Selector1/1 -> Reshape/1  "<p_return>"

== system FMS22/FMS Commander/Arm/SubMode/Return/Heading Commander ==
  FMS_In : Inport
  p1p2 : Inport  Port=2
  Heading Control : Subsystem
  Included Angle : Subsystem
  North : Constant  Value=[1 0]  OutDataTypeStr=single
  psi_rad_cmd : Outport
  wires:
  p1p2/1 -> Included Angle/2(vec2)
  FMS_In/1 -> Heading Control/1(FMS_In)
  North/1 -> Included Angle/1(vec1)
  Included Angle/1(angle_rad) -> Heading Control/2(psi_cmd_rad)
  Heading Control/1(psi_rate_cmd_radPs) -> psi_rad_cmd/1

== system FMS22/FMS Commander/Arm/SubMode/Return/Velocity Commander ==
  p1 : Inport
  p2 : Inport  Port=2
  p3 : Inport  Port=3
  L1 : Inport  Port=4
  In Bus Element : Inport  Port=5  PortName=INS_Out  Element=vn
  In Bus Element1 : Inport  Port=5  PortName=INS_Out  Element=ve
  In Bus Element2 : Inport  Port=5  PortName=INS_Out  Element=psi
  "Cruise Speed " : Subsystem
  Demux : Demux  Outputs=3
  L1 Reference WP : Subsystem
  Lateral Acceleration : Subsystem
  Lateral Acceleration To Speed : Subsystem
  Mux1 : Mux  Inputs=2
  u_cmd : Outport
  v_cmd : Outport  Port=2
  w_cmd : Outport  Port=3
  wires:
  p3/1 -> "Cruise Speed "/1(P2), Lateral Acceleration/3(p3), L1 Reference WP/3(P3)
  In Bus Element1/1 -> Mux1/2
  Mux1/1 -> Lateral Acceleration/1(Vg)
  p2/1 -> "Cruise Speed "/2(P3), Lateral Acceleration To Speed/3(p2), L1 Reference WP/2(P2)
  Demux/2 -> v_cmd/1
  Demux/3 -> w_cmd/1
  Demux/1 -> u_cmd/1
  In Bus Element/1 -> Mux1/1
  L1 Reference WP/1(L1_WP) -> Lateral Acceleration/2(L1_WP)  "L1_WP"
  p1/1 -> Lateral Acceleration To Speed/2(p1), L1 Reference WP/1(P1)
  L1/1 -> Lateral Acceleration/4(L1), L1 Reference WP/4(L1)
  Lateral Acceleration/1(l1_a_cmd) -> Lateral Acceleration To Speed/1(l1_a)
  In Bus Element2/1 -> Lateral Acceleration To Speed/5(psi)
  "Cruise Speed "/1(|Vg|) -> Lateral Acceleration To Speed/4(|Vg|)
  Lateral Acceleration To Speed/1(Vg_C_cmd) -> Demux/1

== system FMS22/FMS Commander/Arm/SubMode/Takeoff/Hold Position ==
  FMS_In : Inport
  Bus Selector : BusSelector  OutputSignals=INS_Out.psi
  Bus Selector1 : BusSelector  OutputSignals=Cmd_In.p_takeoff
  Bus_Selection : Subsystem
  Constant : Constant  Value=0  OutDataTypeStr=Inherit: Inherit via back propagation
  Gain2 : Gain  Gain=FMS_PARAM.XY_P  OutDataTypeStr=single
  Multiply : Product  Multiplication=Matrix(*)
  Mux : Mux  Inputs=2
  Psi To DCM : FMT_Model_Lib/Transformation/Psi To DCM
      settings: SourceProductName=FMT Toolbox
  Reshape : Reshape  OutputDimensionality=Customize  OutputDimensions=[2,1]
  Saturation1 : Saturate  UpperLimit=FMS_PARAM.VEL_XY_LIM/5  LowerLimit=-FMS_PARAM.VEL_XY_LIM/5
  Selector : Selector  InputPortWidth=3  IndexOptions=Index vector (dialog)  Indices=[1 2]  OutputSizes=1
  Sum : Sum  Inputs=-+|
  uv_cmd_mPs : Outport
  wires:
  Reshape/1 -> Sum/2
  Saturation1/1 -> uv_cmd_mPs/1
  Bus Selector/1 -> Psi To DCM/1  "<psi>"
  Selector/1 -> Gain2/1
  Mux/1 -> Multiply/2
  Multiply/1 -> Selector/1
  Psi To DCM/1 -> Multiply/1  "M_CO"
  Constant/1 -> Mux/2
  FMS_In/1 -> Bus Selector1/1, Bus_Selection/1(FMS_In), Bus Selector/1
  Sum/1 -> Mux/1  "xy_err_R"
  Bus_Selection/1(xy_R_O_m) -> Sum/1  "xy_est_R"
  Gain2/1 -> Saturation1/1
  Bus Selector1/1 -> Reshape/1  "<p_takeoff>"

== system FMS22/FMS Commander/Arm/Assist/Altitude/Altitude Command/Controller ==
  motion_state : Inport
  In Bus Element : Inport  Port=2  PortName=FMS_In
  In Bus Element1 : Inport  Port=2  PortName=FMS_In
  Brake Control : Subsystem  TreatAsAtomicUnit=on
  Hold Control : Subsystem  TreatAsAtomicUnit=on
  Merge : Merge  Inputs=3
  Move Control : Subsystem  TreatAsAtomicUnit=on
  Saturation1 : Saturate  UpperLimit=FMS_PARAM.VEL_Z_LIM  LowerLimit=-FMS_PARAM.VEL_Z_LIM
  Switch Case : SwitchCase  CaseConditions={MotionState.Hold, MotionState.Brake, MotionState.Move}  ShowDefaultCase=off
  w_cmd_mPs : Outport
  wires:
  Move Control/1(w_cmd_mPs) -> Merge/3
  Brake Control/1(psi_rate_cmd_radPs) -> Merge/2
  Hold Control/1(w_cmd_mPs) -> Merge/1
  In Bus Element/1 -> Hold Control/1(FMS_In)
  Switch Case/3 -> Move Control/Action
  Switch Case/2 -> Brake Control/Action
  Switch Case/1 -> Hold Control/Action
  motion_state/1 -> Switch Case/1
  Saturation1/1 -> w_cmd_mPs/1
  Merge/1 -> Saturation1/1
  In Bus Element1/1 -> Move Control/1(FMS_In)

== system FMS22/FMS Commander/Arm/Assist/Altitude/Altitude Command/Detect Movement ==
  FMS_In : Inport
  Abs : Abs
  Abs1 : Abs
  Bus Selector : BusSelector  OutputSignals=Pilot_Cmd.stick_throttle,INS_Out.vd
  Compare To Constant : simulink/Logic and Bit Operations/Compare To Constant  relop=>  const=FMS_PARAM.THROTTLE_DZ  OutDataTypeStr=boolean
  Motion Status : Stateflow chart  TreatAsAtomicUnit=on
  motion_state : Outport
  wires:
  FMS_In/1 -> Bus Selector/1
  Abs1/1 -> Compare To Constant/1
  Motion Status/1(state) -> motion_state/1
  Compare To Constant/1 -> Motion Status/1(motion_req)
  Abs/1 -> Motion Status/2(speed)
  Bus Selector/1 -> Abs1/1  "<stick_throttle>"
  Bus Selector/2 -> Abs/1  "<vd>"

== system FMS22/FMS Commander/Arm/Assist/Altitude/Attitude Command/DeadZone ==
  u : Inport
  Dead Zone : DeadZone  LowerValue=-th  UpperValue=th  SaturateOnIntegerOverflow=on
  Gain : Gain  Gain=1/(1-th)
  y : Outport
  wires:
  Gain/1 -> y/1
  Dead Zone/1 -> Gain/1
  u/1 -> Dead Zone/1

== system FMS22/FMS Commander/Arm/Assist/Altitude/Attitude Command/DeadZone2 ==
  u : Inport
  Dead Zone : DeadZone  LowerValue=-th  UpperValue=th  SaturateOnIntegerOverflow=on
  Gain : Gain  Gain=1/(1-th)
  y : Outport
  wires:
  u/1 -> Dead Zone/1
  Dead Zone/1 -> Gain/1
  Gain/1 -> y/1

== system FMS22/FMS Commander/Arm/Assist/Altitude/Attitude Command/Phi_CMD_TD ==
  v : Inport
  Integrator : DiscreteIntegrator  SampleTime=-1  ICPrevOutput=DiscIntNeverNeededParam  ICPrevScaledInput=DiscIntNeverNeededParam
  Integrator1 : DiscreteIntegrator  SampleTime=-1  ICPrevOutput=DiscIntNeverNeededParam  ICPrevScaledInput=DiscIntNeverNeededParam
  Subtract : Sum  Inputs=+-
  "fhan " : Subsystem  mask{r0=4*pi, h0=0.04}
      mask DialogControl ParameterGroupVar Prompt: fhan(v1,v2,r0,h0)
  v1 : Outport
  wires:
  "fhan "/1(fhan) -> Integrator/1
  Subtract/1 -> "fhan "/1(v1)
  Integrator/1 -> Integrator1/1, "fhan "/2(v2)  "v2"
  v/1 -> Subtract/2
  Integrator1/1 -> Subtract/1, v1/1

== system FMS22/FMS Commander/Arm/Assist/Altitude/Attitude Command/Theta_CMD_TD ==
  v : Inport
  Integrator : DiscreteIntegrator  SampleTime=-1  ICPrevOutput=DiscIntNeverNeededParam  ICPrevScaledInput=DiscIntNeverNeededParam
  Integrator1 : DiscreteIntegrator  SampleTime=-1  ICPrevOutput=DiscIntNeverNeededParam  ICPrevScaledInput=DiscIntNeverNeededParam
  Subtract : Sum  Inputs=+-
  "fhan " : Subsystem  mask{r0=4*pi, h0=0.04}
      mask DialogControl ParameterGroupVar Prompt: fhan(v1,v2,r0,h0)
  v1 : Outport
  wires:
  Integrator1/1 -> v1/1, Subtract/1
  v/1 -> Subtract/2
  Integrator/1 -> Integrator1/1, "fhan "/2(v2)  "v2"
  Subtract/1 -> "fhan "/1(v1)
  "fhan "/1(fhan) -> Integrator/1

== system FMS22/FMS Commander/Arm/Assist/Altitude/Heading Command/Controller ==
  motion_state : Inport
  In Bus Element : Inport  Port=2  PortName=FMS_In
  In Bus Element1 : Inport  Port=2  PortName=FMS_In
  Brake Control : Subsystem  TreatAsAtomicUnit=on
  Hold Control : Subsystem  TreatAsAtomicUnit=on
  Merge : Merge  Inputs=3
  Move Control : Subsystem  TreatAsAtomicUnit=on
  Saturation : Saturate  UpperLimit=FMS_PARAM.YAW_RATE_LIM  LowerLimit=-FMS_PARAM.YAW_RATE_LIM
  Switch Case : SwitchCase  CaseConditions={MotionState.Hold, MotionState.Brake, MotionState.Move}  ShowDefaultCase=off
  psi_rate_cmd_radPs : Outport
  wires:
  Move Control/1(psi_rate_cmd_radPs) -> Merge/3
  Brake Control/1(psi_rate_cmd_radPs) -> Merge/2
  Hold Control/1(psi_rate_cmd_radPs) -> Merge/1
  In Bus Element/1 -> Hold Control/1(FMS_In)
  Switch Case/3 -> Move Control/Action
  Switch Case/2 -> Brake Control/Action
  Switch Case/1 -> Hold Control/Action
  motion_state/1 -> Switch Case/1
  Saturation/1 -> psi_rate_cmd_radPs/1
  Merge/1 -> Saturation/1
  In Bus Element1/1 -> Move Control/1(FMS_In)

== system FMS22/FMS Commander/Arm/Assist/Altitude/Heading Command/Detect Movement ==
  FMS_In : Inport
  Abs : Abs
  Abs1 : Abs
  Bus Selector : BusSelector  OutputSignals=Pilot_Cmd.stick_yaw,INS_Out.r
  Compare To Constant : simulink/Logic and Bit Operations/Compare To Constant  relop=>  const=FMS_PARAM.YAW_DZ  OutDataTypeStr=boolean
  Motion State : Stateflow chart  TreatAsAtomicUnit=on
  motion_state : Outport
  wires:
  FMS_In/1 -> Bus Selector/1
  Abs1/1 -> Compare To Constant/1
  Motion State/1(state) -> motion_state/1
  Compare To Constant/1 -> Motion State/1(motion_req)
  Abs/1 -> Motion State/2(speed)
  Bus Selector/1 -> Abs1/1  "<stick_yaw>"
  Bus Selector/2 -> Abs/1  "<r>"

== system FMS22/FMS Commander/Arm/Assist/Position/Altitude Command/Controller ==
  motion_state : Inport
  In Bus Element : Inport  Port=2  PortName=FMS_In
  In Bus Element1 : Inport  Port=2  PortName=FMS_In
  Brake Control : Subsystem  TreatAsAtomicUnit=on
  Hold Control : Subsystem  TreatAsAtomicUnit=on
  Merge : Merge  Inputs=3
  Move Control : Subsystem  TreatAsAtomicUnit=on
  Saturation1 : Saturate  UpperLimit=FMS_PARAM.VEL_Z_LIM  LowerLimit=-FMS_PARAM.VEL_Z_LIM
  Switch Case : SwitchCase  CaseConditions={MotionState.Hold, MotionState.Brake, MotionState.Move}  ShowDefaultCase=off
  w_cmd_mPs : Outport
  wires:
  Move Control/1(w_cmd_mPs) -> Merge/3
  Brake Control/1(psi_rate_cmd_radPs) -> Merge/2
  Hold Control/1(w_cmd_mPs) -> Merge/1
  In Bus Element/1 -> Hold Control/1(FMS_In)
  Switch Case/3 -> Move Control/Action
  Switch Case/2 -> Brake Control/Action
  Switch Case/1 -> Hold Control/Action
  motion_state/1 -> Switch Case/1
  Saturation1/1 -> w_cmd_mPs/1
  Merge/1 -> Saturation1/1
  In Bus Element1/1 -> Move Control/1(FMS_In)

== system FMS22/FMS Commander/Arm/Assist/Position/Altitude Command/Detect Movement ==
  FMS_In : Inport
  Abs : Abs
  Abs1 : Abs
  Bus Selector : BusSelector  OutputSignals=Pilot_Cmd.stick_throttle,INS_Out.vd
  Compare To Constant : simulink/Logic and Bit Operations/Compare To Constant  relop=>  const=FMS_PARAM.THROTTLE_DZ  OutDataTypeStr=boolean
  Motion Status : Stateflow chart  TreatAsAtomicUnit=on
  motion_state : Outport
  wires:
  FMS_In/1 -> Bus Selector/1
  Abs1/1 -> Compare To Constant/1
  Motion Status/1(state) -> motion_state/1
  Compare To Constant/1 -> Motion Status/1(motion_req)
  Abs/1 -> Motion Status/2(speed)
  Bus Selector/1 -> Abs1/1  "<stick_throttle>"
  Bus Selector/2 -> Abs/1  "<vd>"

== system FMS22/FMS Commander/Arm/Assist/Position/Heading Command/Controller ==
  motion_state : Inport
  In Bus Element : Inport  Port=2  PortName=FMS_In
  In Bus Element1 : Inport  Port=2  PortName=FMS_In
  Brake Control : Subsystem  TreatAsAtomicUnit=on
  Hold Control : Subsystem  TreatAsAtomicUnit=on
  Merge : Merge  Inputs=3
  Move Control : Subsystem  TreatAsAtomicUnit=on
  Saturation : Saturate  UpperLimit=FMS_PARAM.YAW_RATE_LIM  LowerLimit=-FMS_PARAM.YAW_RATE_LIM
  Switch Case : SwitchCase  CaseConditions={MotionState.Hold, MotionState.Brake, MotionState.Move}  ShowDefaultCase=off
  psi_rate_cmd_radPs : Outport
  wires:
  Move Control/1(psi_rate_cmd_radPs) -> Merge/3
  Brake Control/1(psi_rate_cmd_radPs) -> Merge/2
  Hold Control/1(psi_rate_cmd_radPs) -> Merge/1
  In Bus Element/1 -> Hold Control/1(FMS_In)
  Switch Case/3 -> Move Control/Action
  Switch Case/2 -> Brake Control/Action
  Switch Case/1 -> Hold Control/Action
  motion_state/1 -> Switch Case/1
  Saturation/1 -> psi_rate_cmd_radPs/1
  Merge/1 -> Saturation/1
  In Bus Element1/1 -> Move Control/1(FMS_In)
